simulink model "sync_subsystem_example"  (R2019b)
settings: Solver=FixedStepDiscrete  StartTime=0.0  StopTime=10.0  RelTol=1e-3
libraries: hdlsllib x1, simulink x1
settings Model: DataTypeOverride=Off  Creator=cchung  LastModifiedBy=bhisma
settings DataIOCC: SaveOutput=off  SaveTime=off  ReturnWorkspaceOutputs=off
settings OptimizationCC: BlockReduction=off  ConditionallyExecuteInputs=off  DefaultParameterBehavior=Inlined
settings DebuggingCC: AlgebraicLoopMsg=error  SingleTaskRateTransMsg=error  StrictBusMsg=ErrorOnBusTreatedAsVector  ArithmeticOperatorsInVariantConditions=warning
settings HardwareCC: ProdBitPerPointer=32  ProdBitPerSizeT=32  ProdBitPerPtrDiffT=32  ProdLargestAtomicFloat=None  ProdIntDivRoundTo=Undefined  ProdEndianess=Unspecified  ProdWordSize=32  ProdHWDeviceType=ASIC/FPGA->ASIC/FPGA  ProdEqTarget=off
settings SFSimCC: SimUseLocalCustomCode=off  CustomCodeUndefinedFunction=UseInterfaceOnly
settings RTWCC: RTWUseLocalCustomCode=off
settings CodeAppCC: StateflowObjectComments=on

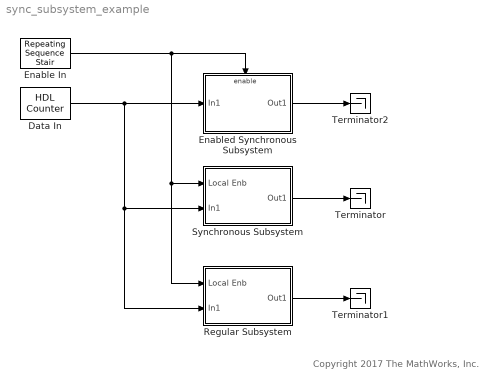
== system sync_subsystem_example ==
  note: Copyright 2017 The MathWorks, Inc.
  Data In : hdlsllib/Sources/HDL Counter  CountType=Free running  CountInit=0  CountStep=1  CountMax=25  CountFromType=Initial value  CountFrom=0  CountResetPort=off  CountLoadPort=off  CountEnbPort=off  CountDirPort=off  CountDataType=Unsigned  CountWordLen=8  CountFracLen=0  CountSampTime=1
      settings: SourceProductName=Simulink
  Enable In : simulink/Sources/Repeating Sequence Stair  OutValues=[0 1 0 0 1 1 0 0]  tsamp=1  OutMin=[]  OutMax=[]  OutDataTypeStr=fixdt('boolean')  OutputDataTypeScalingMode=Specify via dialog  OutDataType=fixdt('boolean')  ConRadixGroup=Best Precision: Vector-wise  OutScaling=[]
  Enabled Synchronous Subsystem : Subsystem  TreatAsAtomicUnit=on
  Regular Subsystem : Subsystem
  Synchronous Subsystem : Subsystem
  Terminator : Terminator
  Terminator1 : Terminator
  Terminator2 : Terminator
  wires:
  Data In/1 -> Regular Subsystem/2(In1), Synchronous Subsystem/2(In1), Enabled Synchronous Subsystem/1(In1)
  Synchronous Subsystem/1(Out1) -> Terminator/1
  Regular Subsystem/1(Out1) -> Terminator1/1
  Enable In/1 -> Regular Subsystem/1(Local Enb), Synchronous Subsystem/1(Local Enb), Enabled Synchronous Subsystem/Enable
  Enabled Synchronous Subsystem/1(Out1) -> Terminator2/1

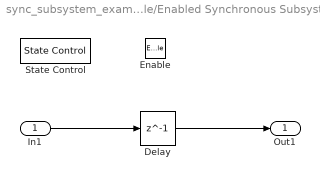
== system sync_subsystem_example/Enabled Synchronous Subsystem ==
  In1 : Inport
  Enable : EnablePort
  Delay : Delay  DelayLength=1
  State Control : StateControl  StateControl=Synchronous
  Out1 : Outport
  wires:
  In1/1 -> Delay/1
  Delay/1 -> Out1/1

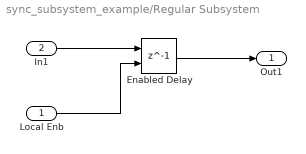
== system sync_subsystem_example/Regular Subsystem ==
  Local Enb : Inport
  In1 : Inport  Port=2
  Enabled Delay : Delay  DelayLength=1  ShowEnablePort=on
      settings: InputPortMap=u0,e6
  Out1 : Outport
  wires:
  In1/1 -> Enabled Delay/1
  Local Enb/1 -> Enabled Delay/2
  Enabled Delay/1 -> Out1/1

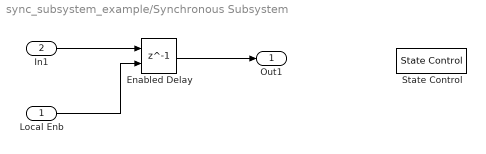
== system sync_subsystem_example/Synchronous Subsystem ==
  Local Enb : Inport
  In1 : Inport  Port=2
  Enabled Delay : Delay  DelayLength=1  ShowEnablePort=on
      settings: InputPortMap=u0,e6
  State Control : StateControl  StateControl=Synchronous
  Out1 : Outport
  wires:
  In1/1 -> Enabled Delay/1
  Local Enb/1 -> Enabled Delay/2
  Enabled Delay/1 -> Out1/1
